simulink model "pipeline15bit_C"  (R2021b)
settings: Solver=VariableStepAuto  StartTime=0.0  StopTime=5000.0  RelTol=1e-3
libraries: simulink x2
settings Model: Creator=DELL  LastModifiedBy=DELL

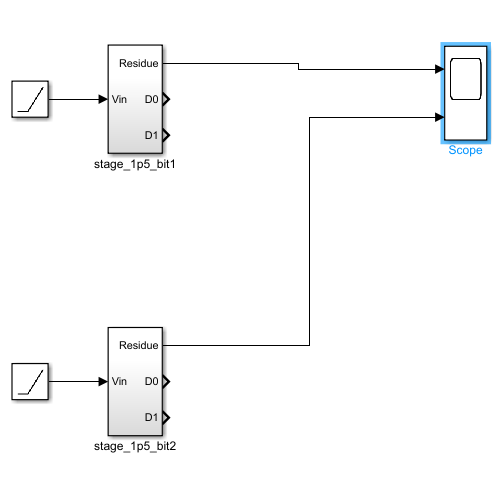
[thumbnail: Simulink's stored preview of the top-level diagram]
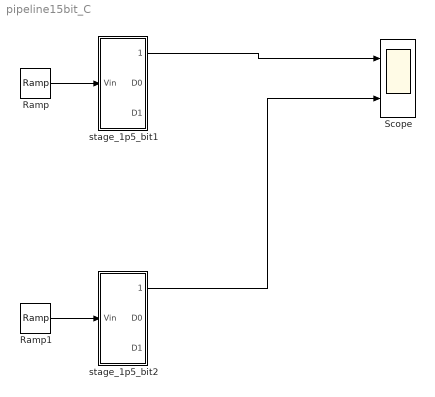
== system pipeline15bit_C ==
  Ramp : simulink/Sources/Ramp  slope=1/160  start=0  InitialOutput=-1
  Ramp1 : simulink/Sources/Ramp  slope=1/160  start=0  InitialOutput=-1
  Scope : Scope  NumInputPorts=2
  stage_1p5_bit1 : Subsystem
  stage_1p5_bit2 : Subsystem
  wires:
  Ramp1/1 -> stage_1p5_bit2/1(Vin)
  Ramp/1 -> stage_1p5_bit1/1(Vin)
  stage_1p5_bit1/1(Residue) -> Scope/1
  stage_1p5_bit2/1(Residue) -> Scope/2

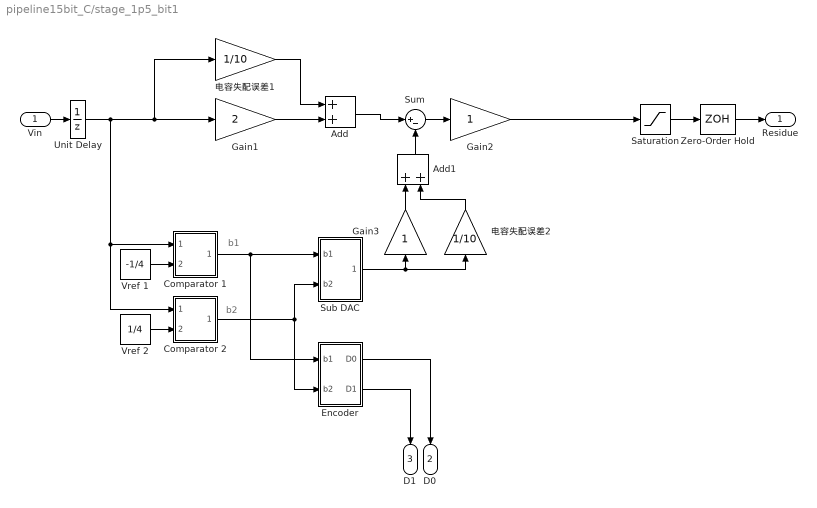
== system pipeline15bit_C/stage_1p5_bit1 ==
  note: b2
  note: b1
  Vin : Inport
  Add : Sum
  Add1 : Sum
  Comparator 1 : Subsystem
  Comparator 2 : Subsystem
  Encoder : Subsystem
  Gain1 : Gain  Gain=2
  Gain2 : Gain
  Gain3 : Gain
  Saturation : Saturate  UpperLimit=1  LowerLimit=-1
  Sub DAC : Subsystem
  Sum : Sum  Inputs=|+-
  Unit Delay : UnitDelay  SampleTime=-1  HasFrameUpgradeWarning=on
  Vref 1 : Constant  Value=-1/4
  Vref 2 : Constant  Value=1/4
  Zero-Order Hold : ZeroOrderHold
  电容失配误差1 : Gain  Gain=1/10
  电容失配误差2 : Gain  Gain=1/10
  Residue : Outport
  D0 : Outport  Port=2
  D1 : Outport  Port=3
  wires:
  Vref 1/1 -> Comparator 1/2(Vref)
  Sum/1 -> Gain2/1
  Saturation/1 -> Zero-Order Hold/1
  Zero-Order Hold/1 -> Residue/1
  Vref 2/1 -> Comparator 2/2(Vref)
  Comparator 2/1(Out) -> Sub DAC/2(b2), Encoder/2(b2)
  Vin/1 -> Unit Delay/1
  Comparator 1/1(Out) -> Encoder/1(b1), Sub DAC/1(b1)
  Unit Delay/1 -> Comparator 1/1(Vin), Comparator 2/1(Vin), 电容失配误差1/1, Gain1/1
  Sub DAC/1(Vdac) -> 电容失配误差2/1, Gain3/1
  Encoder/1(D0) -> D0/1
  Encoder/2(D1) -> D1/1
  Add1/1 -> Sum/2
  Gain3/1 -> Add1/1
  Gain2/1 -> Saturation/1
  Gain1/1 -> Add/2
  Add/1 -> Sum/1
  电容失配误差1/1 -> Add/1
  电容失配误差2/1 -> Add1/2

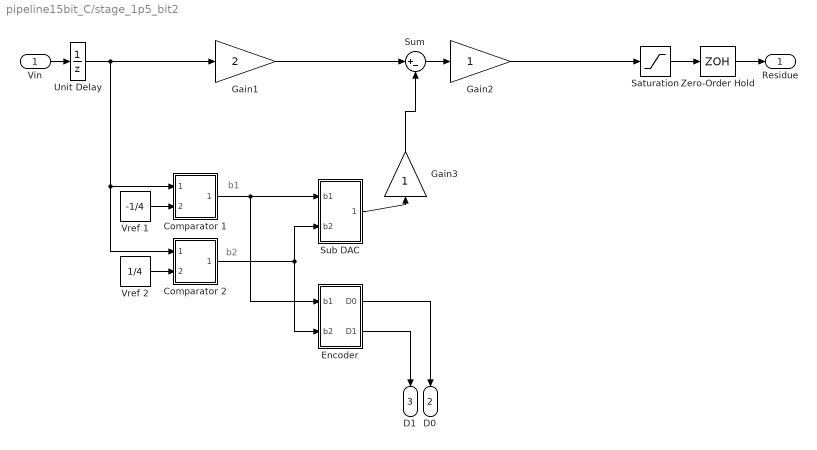
== system pipeline15bit_C/stage_1p5_bit2 ==
  note: b2
  note: b1
  Vin : Inport
  Comparator 1 : Subsystem
  Comparator 2 : Subsystem
  Encoder : Subsystem
  Gain1 : Gain  Gain=2
  Gain2 : Gain
  Gain3 : Gain
  Saturation : Saturate  UpperLimit=1  LowerLimit=-1
  Sub DAC : Subsystem
  Sum : Sum  Inputs=|+-
  Unit Delay : UnitDelay  SampleTime=-1  HasFrameUpgradeWarning=on
  Vref 1 : Constant  Value=-1/4
  Vref 2 : Constant  Value=1/4
  Zero-Order Hold : ZeroOrderHold
  Residue : Outport
  D0 : Outport  Port=2
  D1 : Outport  Port=3
  wires:
  Vref 1/1 -> Comparator 1/2(Vref)
  Sum/1 -> Gain2/1
  Saturation/1 -> Zero-Order Hold/1
  Zero-Order Hold/1 -> Residue/1
  Vref 2/1 -> Comparator 2/2(Vref)
  Comparator 2/1(Out) -> Sub DAC/2(b2), Encoder/2(b2)
  Vin/1 -> Unit Delay/1
  Comparator 1/1(Out) -> Encoder/1(b1), Sub DAC/1(b1)
  Unit Delay/1 -> Comparator 1/1(Vin), Comparator 2/1(Vin), Gain1/1
  Sub DAC/1(Vdac) -> Gain3/1
  Encoder/1(D0) -> D0/1
  Encoder/2(D1) -> D1/1
  Gain3/1 -> Sum/2
  Gain2/1 -> Saturation/1
  Gain1/1 -> Sum/1

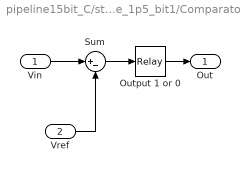
== system pipeline15bit_C/stage_1p5_bit1/Comparator 1 ==
  Vin : Inport
  Vref : Inport  Port=2
  Output 1 or 0 : Relay  OnSwitchValue=0  OffSwitchValue=0
  Sum : Sum  Inputs=|+-
  Out : Outport
  wires:
  Sum/1 -> Output 1 or 0/1
  Vin/1 -> Sum/1
  Output 1 or 0/1 -> Out/1
  Vref/1 -> Sum/2

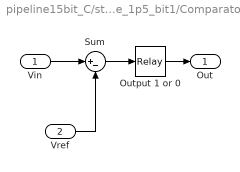
== system pipeline15bit_C/stage_1p5_bit1/Comparator 2 ==
  Vin : Inport
  Vref : Inport  Port=2
  Output 1 or 0 : Relay  OnSwitchValue=0  OffSwitchValue=0
  Sum : Sum  Inputs=|+-
  Out : Outport
  wires:
  Sum/1 -> Output 1 or 0/1
  Vin/1 -> Sum/1
  Output 1 or 0/1 -> Out/1
  Vref/1 -> Sum/2

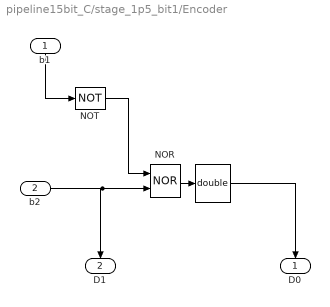
== system pipeline15bit_C/stage_1p5_bit1/Encoder ==
  b1 : Inport
  b2 : Inport  Port=2
  " " : DataTypeConversion  OutDataTypeStr=double
  NOR : Logic  Operator=NOR  AllPortsSameDT=off  OutDataTypeStr=boolean
  NOT : Logic  Operator=NOT  AllPortsSameDT=off  OutDataTypeStr=boolean
  D0 : Outport
  D1 : Outport  Port=2
  wires:
  b2/1 -> D1/1, NOR/2
  NOR/1 -> " "/1
  " "/1 -> D0/1
  NOT/1 -> NOR/1
  b1/1 -> NOT/1

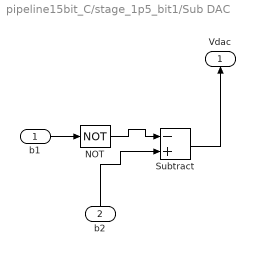
== system pipeline15bit_C/stage_1p5_bit1/Sub DAC ==
  b1 : Inport
  b2 : Inport  Port=2
  NOT : Logic  Operator=NOT  AllPortsSameDT=off  OutDataTypeStr=boolean
  Subtract : Sum  Inputs=-+
  Vdac : Outport
  wires:
  b2/1 -> Subtract/2
  b1/1 -> NOT/1
  Subtract/1 -> Vdac/1
  NOT/1 -> Subtract/1

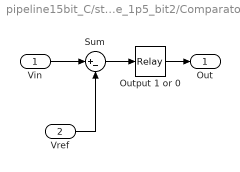
== system pipeline15bit_C/stage_1p5_bit2/Comparator 1 ==
  Vin : Inport
  Vref : Inport  Port=2
  Output 1 or 0 : Relay  OnSwitchValue=0  OffSwitchValue=0
  Sum : Sum  Inputs=|+-
  Out : Outport
  wires:
  Sum/1 -> Output 1 or 0/1
  Vin/1 -> Sum/1
  Output 1 or 0/1 -> Out/1
  Vref/1 -> Sum/2

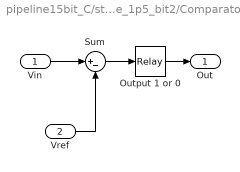
== system pipeline15bit_C/stage_1p5_bit2/Comparator 2 ==
  Vin : Inport
  Vref : Inport  Port=2
  Output 1 or 0 : Relay  OnSwitchValue=0  OffSwitchValue=0
  Sum : Sum  Inputs=|+-
  Out : Outport
  wires:
  Sum/1 -> Output 1 or 0/1
  Vin/1 -> Sum/1
  Output 1 or 0/1 -> Out/1
  Vref/1 -> Sum/2

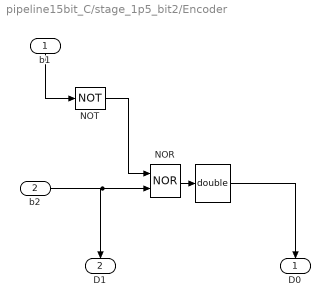
== system pipeline15bit_C/stage_1p5_bit2/Encoder ==
  b1 : Inport
  b2 : Inport  Port=2
  " " : DataTypeConversion  OutDataTypeStr=double
  NOR : Logic  Operator=NOR  AllPortsSameDT=off  OutDataTypeStr=boolean
  NOT : Logic  Operator=NOT  AllPortsSameDT=off  OutDataTypeStr=boolean
  D0 : Outport
  D1 : Outport  Port=2
  wires:
  b2/1 -> D1/1, NOR/2
  NOR/1 -> " "/1
  " "/1 -> D0/1
  NOT/1 -> NOR/1
  b1/1 -> NOT/1

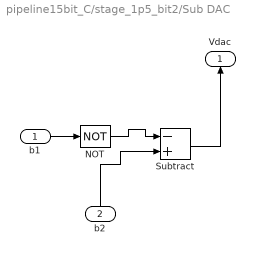
== system pipeline15bit_C/stage_1p5_bit2/Sub DAC ==
  b1 : Inport
  b2 : Inport  Port=2
  NOT : Logic  Operator=NOT  AllPortsSameDT=off  OutDataTypeStr=boolean
  Subtract : Sum  Inputs=-+
  Vdac : Outport
  wires:
  b2/1 -> Subtract/2
  b1/1 -> NOT/1
  Subtract/1 -> Vdac/1
  NOT/1 -> Subtract/1
